simulink model "tut03_1"  (R2026a)
settings: Solver=VariableStepAuto  StopTime=20
settings Model: Creator=vpetrone

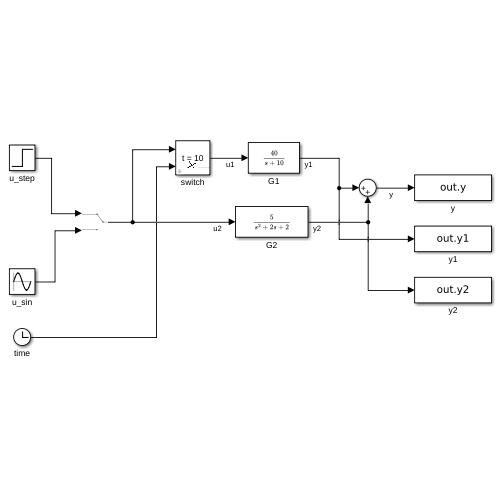
[thumbnail: Simulink's stored preview of the top-level diagram]
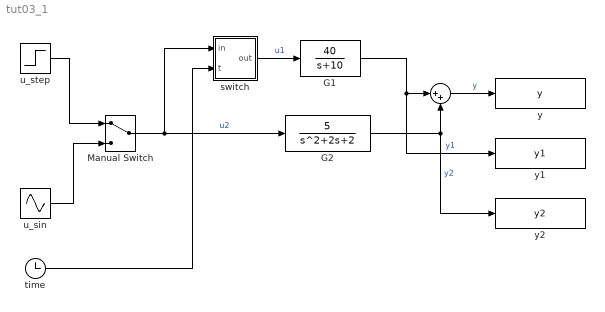
== system tut03_1 ==
  " " : Sum  Inputs=|++
  G1 : TransferFcn  Numerator=[40]  Denominator=[1 10]
  G2 : TransferFcn  Numerator=[5]  Denominator=[1 2 2]
  Manual Switch : ManualSwitch
  switch : Subsystem  Description=Time switch. When the time exceeds the set threshold, the output is 0. Otherwise, the output coincides with the input signal.  mask{T=10}
      mask prompts: T "opening time [s]"
      mask DialogControl DescTextVar Prompt: Time switch. When the time exceeds the set threshold, the output is 0. Otherwise, the output coincides with the input signal.
      mask Display:
      | image('switch.png'); % Use "Edit Image" on toolstrip to change.
      | TT = get_param(gcb, 'opening_time');
      | disp(['t = ' TT])
  time : Clock
  u_sin : Sin  SampleTime=0
  u_step : Step  Time=0  SampleTime=0
  y : ToWorkspace  VariableName=y  SaveFormat=Timeseries  SampleTime=-1
  y1 : ToWorkspace  VariableName=y1  SaveFormat=Timeseries  SampleTime=-1
  y2 : ToWorkspace  VariableName=y2  SaveFormat=Timeseries  SampleTime=-1
  wires:
  G1/1 -> y1/1, " "/1  "y1"
  G2/1 -> y2/1, " "/2  "y2"
  " "/1 -> y/1  "y"
  u_step/1 -> Manual Switch/1
  u_sin/1 -> Manual Switch/2
  switch/1(out) -> G1/1  "u1"
  time/1 -> switch/2(t)
  Manual Switch/1 -> switch/1(in), G2/1  "u2"

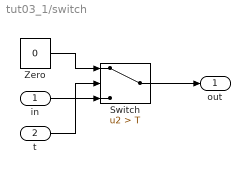
== system tut03_1/switch ==
  in : Inport
  t : Inport  Port=2
  Switch : Switch  Criteria=u2 > Threshold  Threshold=T  SaturateOnIntegerOverflow=off  InputSameDT=off
  Zero : Constant  Value=0  OutDataTypeStr=Inherit: Inherit via back propagation
  out : Outport
  wires:
  Zero/1 -> Switch/1
  Switch/1 -> out/1
  in/1 -> Switch/3
  t/1 -> Switch/2
